simulink model "que7"  (R2020b)
settings: Solver=VariableStepAuto  StartTime=0.0  StopTime=10.0  RelTol=1e-3
settings Model: Creator=ANUJA  LastModifiedBy=ANUJA

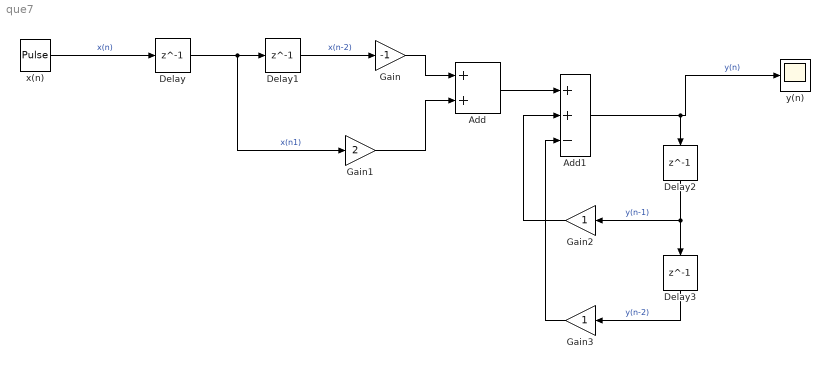
== system que7 ==
  Add : Sum
  Add1 : Sum  Inputs=++-
  Delay{,1..3} (4 alike) : Delay  DelayLength=1  InitialCondition=0
  Gain : Gain  Gain=-1
  Gain1 : Gain  Gain=2
  Gain2 : Gain
  Gain3 : Gain
  x(n) : DiscretePulseGenerator  PulseType=Time based  Period=10  PulseWidth=5
  y(n) : Scope
  wires:
  x(n)/1 -> Delay/1  "x(n)"
  Delay/1 -> Gain1/1, Delay1/1  "x(n1)"
  Delay1/1 -> Gain/1  "x(n-2)"
  Gain/1 -> Add/1
  Gain1/1 -> Add/2
  Add/1 -> Add1/1
  Add1/1 -> y(n)/1, Delay2/1  "y(n)"
  Delay2/1 -> Gain2/1, Delay3/1  "y(n-1)"
  Delay3/1 -> Gain3/1  "y(n-2)"
  Gain3/1 -> Add1/3
  Gain2/1 -> Add1/2
